simulink model "model_sinusoidal_gust"  (R2020b)
settings: configuration reference "Configuration" (kept outside this file)
undefined symbols (not defined in the file or in its folder): CHORD_LENGTH
settings Model: Creator=C:\Users\Dogukan  LastModifiedBy=dogukan
settings ConfigSetRef: SourceName=Configuration  SourceLocation=Base Workspace

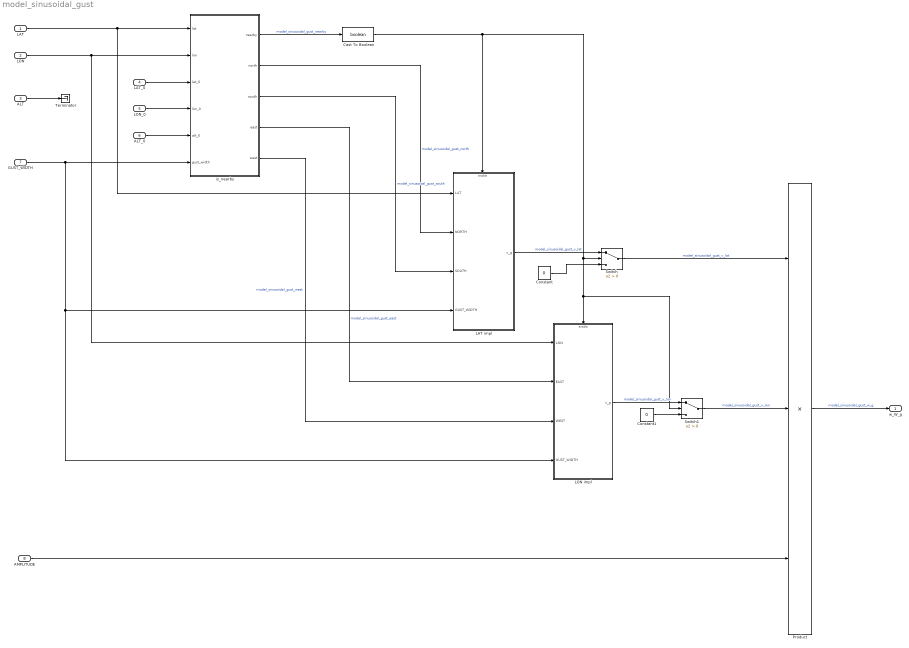
== system model_sinusoidal_gust ==
  LAT : Inport  OutDataTypeStr=double
  LON : Inport  Port=2  OutDataTypeStr=double
  ALT : Inport  Port=3  OutDataTypeStr=double
  LAT_0 : Inport  Port=4  OutDataTypeStr=double
  LON_0 : Inport  Port=5  OutDataTypeStr=double
  ALT_0 : Inport  Port=6  OutDataTypeStr=double
  GUST_WIDTH : Inport  Port=7  OutDataTypeStr=double
  AMPLITUDE : Inport  Port=8  OutDataTypeStr=double
  Cast To Boolean : DataTypeConversion  OutDataTypeStr=boolean
  Constant : Constant  Value=0
  Constant1 : Constant  Value=0
  LAT impl : Subsystem  TreatAsAtomicUnit=on
  LON impl : Subsystem  TreatAsAtomicUnit=on
  Product : Product  Inputs=3
  Switch : Switch  Criteria=u2 > Threshold
  Switch1 : Switch  Criteria=u2 > Threshold
  Terminator : Terminator
  is_nearby : MATLAB Function  TreatAsAtomicUnit=on
  w_W_g : Outport  OutDataTypeStr=double
  wires:
  LAT/1 -> is_nearby/1(lat), LAT impl/1(LAT)
  LON/1 -> LON impl/1(LON), is_nearby/2(lon)
  LAT_0/1 -> is_nearby/3(lat_0)
  LON_0/1 -> is_nearby/4(lon_0)
  ALT_0/1 -> is_nearby/5(alt_0)
  GUST_WIDTH/1 -> LON impl/4(GUST_WIDTH), LAT impl/4(GUST_WIDTH), is_nearby/6(gust_width)
  AMPLITUDE/1 -> Product/3
  is_nearby/1(nearby) -> Cast To Boolean/1  "model_sinusoidal_gust_nearby"
  is_nearby/2(north) -> LAT impl/2(NORTH)  "model_sinusoidal_gust_north"
  is_nearby/3(south) -> LAT impl/3(SOUTH)  "model_sinusoidal_gust_south"
  is_nearby/4(east) -> LON impl/2(EAST)  "model_sinusoidal_gust_east"
  is_nearby/5(west) -> LON impl/3(WEST)  "model_sinusoidal_gust_west"
  Switch/1 -> Product/1  "model_sinusoidal_gust_v_lat"
  Switch1/1 -> Product/2  "model_sinusoidal_gust_v_lon"
  Product/1 -> w_W_g/1  "model_sinusoidal_gust_w_g"
  Cast To Boolean/1 -> Switch1/2, LON impl/Enable, Switch/2, LAT impl/Enable
  Constant/1 -> Switch/3
  LAT impl/1(v_g) -> Switch/1  "model_sinusoidal_gust_v_lat"
  Constant1/1 -> Switch1/3
  LON impl/1(v_g) -> Switch1/1  "model_sinusoidal_gust_v_lon"
  ALT/1 -> Terminator/1

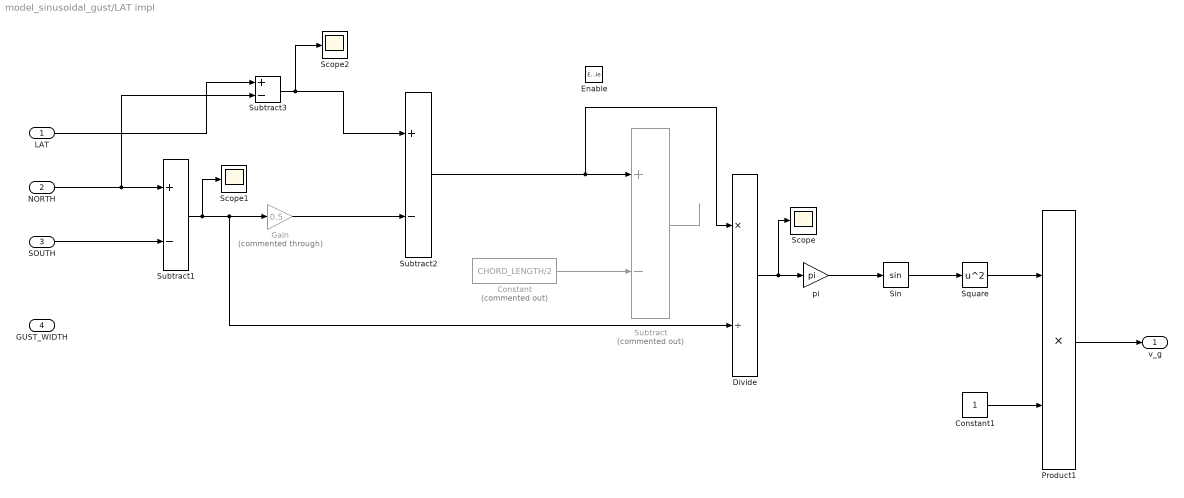
== system model_sinusoidal_gust/LAT impl ==
  LAT : Inport  OutDataTypeStr=double
  NORTH : Inport  Port=2  OutDataTypeStr=double
  SOUTH : Inport  Port=3  OutDataTypeStr=double
  GUST_WIDTH : Inport  Port=4  OutDataTypeStr=double
  Enable : EnablePort
  Constant : Constant  Commented=on  Value=CHORD_LENGTH/2
  Constant1 : Constant
  Divide : Product  Inputs=*/
  Gain : Gain  Commented=through  Gain=0.5
  Product1 : Product
  Scope : Scope
  Scope1 : Scope
  Scope2 : Scope
  Sin : Trigonometry
  Square : Math  Operator=square  SaturateOnIntegerOverflow=on
  Subtract : Sum  Commented=on  Inputs=+-
  Subtract1 : Sum  Inputs=+-
  Subtract2 : Sum  Inputs=+-
  Subtract3 : Sum  Inputs=+-
  pi : Gain  Gain=pi
  v_g : Outport  OutDataTypeStr=double
  wires:
  Divide/1 -> Scope/1, pi/1
  pi/1 -> Sin/1
  Square/1 -> Product1/1
  Sin/1 -> Square/1
  Product1/1 -> v_g/1
  Constant/1 -> Subtract/2
  Subtract/1 -> ?
  NORTH/1 -> Subtract1/1, Subtract3/2
  SOUTH/1 -> Subtract1/2
  Subtract1/1 -> Scope1/1, Gain/1, Divide/2
  LAT/1 -> Subtract3/1
  Subtract2/1 -> Subtract/1, Divide/1
  Gain/1 -> Subtract2/2
  Subtract3/1 -> Scope2/1, Subtract2/1
  Constant1/1 -> Product1/2

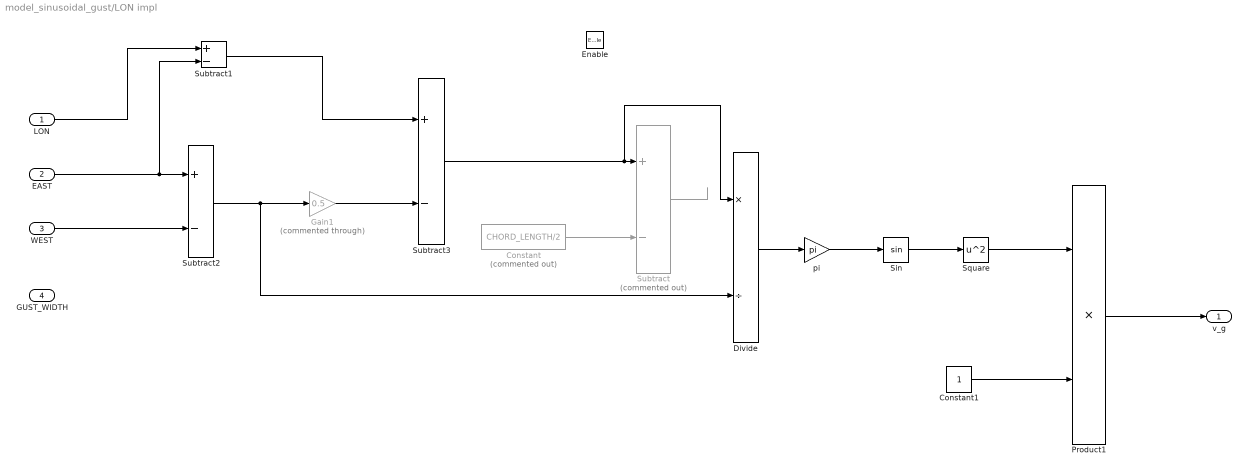
== system model_sinusoidal_gust/LON impl ==
  LON : Inport  OutDataTypeStr=double
  EAST : Inport  Port=2  OutDataTypeStr=double
  WEST : Inport  Port=3  OutDataTypeStr=double
  GUST_WIDTH : Inport  Port=4  OutDataTypeStr=double
  Enable : EnablePort
  Constant : Constant  Commented=on  Value=CHORD_LENGTH/2
  Constant1 : Constant
  Divide : Product  Inputs=*/
  Gain1 : Gain  Commented=through  Gain=0.5
  Product1 : Product
  Sin : Trigonometry
  Square : Math  Operator=square  SaturateOnIntegerOverflow=on
  Subtract : Sum  Commented=on  Inputs=+-
  Subtract1 : Sum  Inputs=+-
  Subtract2 : Sum  Inputs=+-
  Subtract3 : Sum  Inputs=+-
  pi : Gain  Gain=pi
  v_g : Outport  OutDataTypeStr=double
  wires:
  Divide/1 -> pi/1
  pi/1 -> Sin/1
  Square/1 -> Product1/1
  Sin/1 -> Square/1
  Product1/1 -> v_g/1
  Subtract/1 -> ?
  Gain1/1 -> Subtract3/2
  Subtract3/1 -> Divide/1, Subtract/1
  LON/1 -> Subtract1/1
  Subtract2/1 -> Divide/2, Gain1/1
  EAST/1 -> Subtract1/2, Subtract2/1
  WEST/1 -> Subtract2/2
  Constant/1 -> Subtract/2
  Constant1/1 -> Product1/2
  Subtract1/1 -> Subtract3/1

== matlab function model_sinusoidal_gust/is_nearby ==
  data: lat input; nearby output; lon input; lat_0 input; lon_0 input; alt_0 input; gust_width input; north output; south output; east output; west output
% model_sinusoidal_gust
function [nearby, north, south, east, west] = is_nearby(lat, lon, lat_0, lon_0, alt_0, gust_width)
    % Units:
    % [lat] = rad
    % [lon] = rad
    % [lat_0] = rad
    % [lon_0] = rad
    % [height_0] = m
    % [gust_width] = m
    % Independet of altitude, phenomena is available on all heights, because otherwise height distribution is needed

    % Option 1: doesn't support code gen
    % [arclen, az] = distance(lat, lon, lat0, lon0);
    % nearby = arclen < width;

    % Option 2: ¯\_(ツ)_/¯
    % earth_radius = 6371000; % m
    % delta_phi = lat - lat_0;
    % delta_lambda = lon - lon_0;
    % a = sin(delta_phi / 2) ^ 2 + cos(lat) * cos(lat_0) * cos(delta_lambda / 2) ^ 2;
    % c = 2 * atan2(sqrt(a), sqrt(1 - a));
    % dist = earth_radius * c;
    % nearby = dist < width;

    % Option 3:
    lat_0 = rad2deg(lat_0); % ned2lla needs lla in degrees
    lon_0 = rad2deg(lon_0); % ned2lla needs lla in degrees

    north_lla = ned2lla([gust_width/2, 0, 0], [lat_0, lon_0, alt_0], "flat");
    north = deg2rad(north_lla(1)); % rad
    south_lla = ned2lla([-gust_width/2, 0, 0], [lat_0, lon_0, alt_0], "flat");
    south = deg2rad(south_lla(1)); % rad
    inside_lat = (south < lat) & (lat < north);
    % disp(inside_lat);

    east_lla = ned2lla([0, gust_width/2, 0], [lat_0, lon_0, alt_0], "flat");
    east = deg2rad(east_lla(2)); % rad
    west_lla = ned2lla([0, -gust_width/2, 0], [lat_0, lon_0, alt_0], "flat");
    west = deg2rad(west_lla(2)); % rad
    inside_lon = (west < lon) & (lon < east);
    % disp(inside_lon);

    nearby = inside_lat & inside_lon;
end
